simulink model "MLIinverter"  (R2019a)
settings: Solver=VariableStepAuto  StartTime=0.0  StopTime=10.0  RelTol=1e-3
libraries: powerlib x47, powerlib_meascontrol x15
settings Model: Creator=Administrator  LastModifiedBy=Administrator

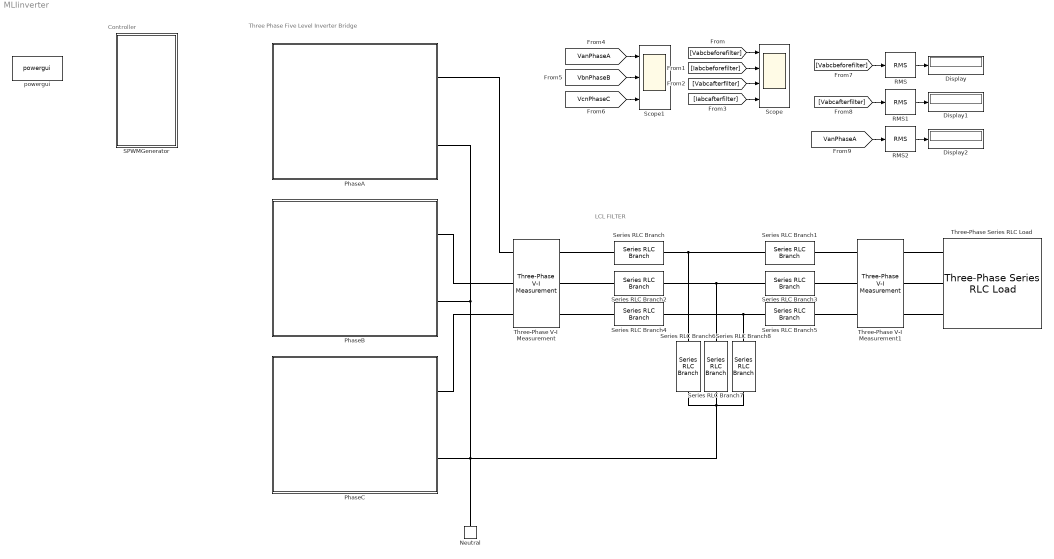
== system MLIinverter ==
  note: LCL FILTER
  note: Controller
  note: Three Phase Five Level Inverter Bridge
  Display : Display
  Display1 : Display
  Display2 : Display
  Neutral : powerlib/Elements/Neutral  LConnTagsString=a  NodeNumber=10
      settings: SourceProductName=Simscape Electrical  SourceProductBaseCode=PS
  PhaseA : Subsystem
  PhaseB : Subsystem
  PhaseC : Subsystem
  RMS : powerlib_meascontrol/Measurements/RMS  TrueRMS=on  Freq=50  RMSInit=0  Ts=0
      settings: SourceProductName=Simscape Electrical
  RMS1 : powerlib_meascontrol/Measurements/RMS  TrueRMS=on  Freq=50  RMSInit=0  Ts=0
      settings: SourceProductName=Simscape Electrical
  RMS2 : powerlib_meascontrol/Measurements/RMS  TrueRMS=on  Freq=50  RMSInit=0  Ts=0
      settings: SourceProductName=Simscape Electrical
  SPWMGenerator : Subsystem
  Scope : Scope  NumInputPorts=4
  Scope1 : Scope  NumInputPorts=3
  Series RLC Branch : powerlib/Elements/Series RLC Branch  LConnTagsString=__new0  RConnTagsString=__new0  BranchType=L  Resistance=1  Inductance=260e-3  SetiL0=off  InitialCurrent=0  Capacitance=1e-6  Setx0=off  InitialVoltage=0  Measurements=None
      settings: SourceProductName=Simscape Electrical
  Series RLC Branch1 : powerlib/Elements/Series RLC Branch  LConnTagsString=__new0  RConnTagsString=__new0  BranchType=L  Resistance=1  Inductance=14e-3  SetiL0=off  InitialCurrent=0  Capacitance=1e-6  Setx0=off  InitialVoltage=0  Measurements=None
      settings: SourceProductName=Simscape Electrical
  Series RLC Branch2 : powerlib/Elements/Series RLC Branch  LConnTagsString=__new0  RConnTagsString=__new0  BranchType=L  Resistance=1  Inductance=260e-3  SetiL0=off  InitialCurrent=0  Capacitance=1e-6  Setx0=off  InitialVoltage=0  Measurements=None
      settings: SourceProductName=Simscape Electrical
  Series RLC Branch3 : powerlib/Elements/Series RLC Branch  LConnTagsString=__new0  RConnTagsString=__new0  BranchType=L  Resistance=1  Inductance=14e-3  SetiL0=off  InitialCurrent=0  Capacitance=1e-6  Setx0=off  InitialVoltage=0  Measurements=None
      settings: SourceProductName=Simscape Electrical
  Series RLC Branch4 : powerlib/Elements/Series RLC Branch  LConnTagsString=__new0  RConnTagsString=__new0  BranchType=L  Resistance=1  Inductance=260e-3  SetiL0=off  InitialCurrent=0  Capacitance=1e-6  Setx0=off  InitialVoltage=0  Measurements=None
      settings: SourceProductName=Simscape Electrical
  Series RLC Branch5 : powerlib/Elements/Series RLC Branch  LConnTagsString=__new0  RConnTagsString=__new0  BranchType=L  Resistance=1  Inductance=14e-3  SetiL0=off  InitialCurrent=0  Capacitance=1e-6  Setx0=off  InitialVoltage=0  Measurements=None
      settings: SourceProductName=Simscape Electrical
  Series RLC Branch6 : powerlib/Elements/Series RLC Branch  LConnTagsString=__new0  RConnTagsString=__new0  BranchType=C  Resistance=1  Inductance=1e-3  SetiL0=off  InitialCurrent=0  Capacitance=18e-6  Setx0=off  InitialVoltage=0  Measurements=None
      settings: SourceProductName=Simscape Electrical
  Series RLC Branch7 : powerlib/Elements/Series RLC Branch  LConnTagsString=__new0  RConnTagsString=__new0  BranchType=C  Resistance=1  Inductance=1e-3  SetiL0=off  InitialCurrent=0  Capacitance=18e-6  Setx0=off  InitialVoltage=0  Measurements=None
      settings: SourceProductName=Simscape Electrical
  Series RLC Branch8 : powerlib/Elements/Series RLC Branch  LConnTagsString=__new0  RConnTagsString=__new0  BranchType=C  Resistance=1  Inductance=1e-3  SetiL0=off  InitialCurrent=0  Capacitance=18e-6  Setx0=off  InitialVoltage=0  Measurements=None
      settings: SourceProductName=Simscape Electrical
  Three-Phase Series RLC Load : powerlib/Elements/Three-Phase Series RLC Load  LConnTagsString=A|B|C  Configuration=Y (grounded)  NominalVoltage=400  Vabc=[1e3 1e3 1e3]  Vabcp=[1e3 1e3 1e3]  NominalFrequency=50  UnbalancedPower=off  ActivePower=1e3  InductivePower=0  CapacitivePower=0  Pabc=[10e3 9e3 11e3]  QLabc=[100 90 110]  QCabc=[100 90 110]  Pabcp=[10e3 9e3 11e3]  QLabcp=[100 90 110]  QCabcp=[100 90 110]  Measurements=None  LoadType=constant PQ
      settings: SourceProductName=Simscape Electrical
  Three-Phase V-I Measurement : powerlib/Measurements/Three-Phase V-I Measurement  VoltageMeasurement=phase-to-phase  SetLabelV=on  LabelV=Vabcbeforefilter  Vpu=off  VpuLL=off  CurrentMeasurement=yes  SetLabelI=on  LabelI=Iabcbeforefilter  Ipu=off  Pbase=100e6  Vbase=500e3  OutputType=Complex  PhasorSimulation=off  PSBequivalent=0
      settings: SourceProductName=Simscape Electrical
  Three-Phase V-I Measurement1 : powerlib/Measurements/Three-Phase V-I Measurement  VoltageMeasurement=phase-to-phase  SetLabelV=on  LabelV=Vabcafterfilter  Vpu=off  VpuLL=off  CurrentMeasurement=yes  SetLabelI=on  LabelI=Iabcafterfilter  Ipu=off  Pbase=100e6  Vbase=500e3  OutputType=Complex  PhasorSimulation=off  PSBequivalent=0
      settings: SourceProductName=Simscape Electrical
  powergui : powerlib/powergui  Priority=1  SimulationMode=Discrete  SampleTime=6e-6  frequency=60  Iterations=50  frequencyindice=0  Pbase=100e6  ErrMax=1e-4  UnitsV=kV  UnitsW=MW  buscounter=0  FunctionMessages=off  echomessages=off  EnableUseOfTLC=off  CurrentSourceSwitches=off  DisableSnubberDevices=off  DisableRonSwitches=off  DisableVfSwitches=off  DisplayEquations=off  AutomaticDiscreteSolvers=off  SolverType=Tustin/Backward Euler (TBE)  Interpol=off  ExternalGateDelay=off  methode=off  Ts=100  x0status=blocks  SPID=on  SwTol=0  HookPort=off  NonlinearTolerance=0  nMaxIteration=15  ContinueOnMaxIteration=off  RestoreLinks=warning  ResistiveCurrentMeasurement=off  Frange=[0:2:500]  Ylog=off  Xlog=on  ShowGrid=off  save=off  variable=ZData  structure=0  ZoomFFT=off  StartTime=0.0  cycles=1  DisplayStyle=1  fundamental=60  FreqAxis=off  MaxFrequency=1000  frequencyindicesteady=1  RmsSteady=1  display=off
      settings: SourceProductName=Simscape Electrical
  wires:
  [Vabcbeforefilter] -> Scope/1
  [Iabcbeforefilter] -> Scope/2
  [Iabcafterfilter] -> Scope/4
  [Vabcafterfilter] -> Scope/3
  [VanPhaseA] -> Scope1/1
  [VbnPhaseB] -> Scope1/2
  [VcnPhaseC] -> Scope1/3
  RMS/1 -> Display/1
  RMS1/1 -> Display1/1
  RMS2/1 -> Display2/1
  [Vabcbeforefilter] -> RMS/1
  [Vabcafterfilter] -> RMS1/1
  [VanPhaseA] -> RMS2/1
  connections:
  PhaseA/RConn1 -- Three-Phase V-I Measurement/LConn1
  PhaseB/RConn1 -- Three-Phase V-I Measurement/LConn2
  PhaseC/RConn1 -- Three-Phase V-I Measurement/LConn3
  Series RLC Branch/LConn1 -- Three-Phase V-I Measurement/RConn1
  Three-Phase V-I Measurement/RConn3 -- Series RLC Branch4/LConn1
  Three-Phase V-I Measurement1/RConn1 -- Three-Phase Series RLC Load/LConn1
  Three-Phase V-I Measurement1/RConn2 -- Three-Phase Series RLC Load/LConn2
  Three-Phase V-I Measurement1/RConn3 -- Three-Phase Series RLC Load/LConn3
  Three-Phase V-I Measurement/RConn2 -- Series RLC Branch2/LConn1
  Series RLC Branch2/RConn1 -- Series RLC Branch7/LConn1 -- Series RLC Branch3/LConn1
  Series RLC Branch1/LConn1 -- Series RLC Branch6/LConn1 -- Series RLC Branch/RConn1
  Series RLC Branch4/RConn1 -- Series RLC Branch5/LConn1 -- Series RLC Branch8/LConn1
  Series RLC Branch3/RConn1 -- Three-Phase V-I Measurement1/LConn2
  Series RLC Branch1/RConn1 -- Three-Phase V-I Measurement1/LConn1
  Three-Phase V-I Measurement1/LConn3 -- Series RLC Branch5/RConn1
  PhaseA/RConn2 -- PhaseB/RConn2 -- Series RLC Branch8/RConn1 -- Series RLC Branch7/RConn1 -- Series RLC Branch6/RConn1 -- Neutral/LConn1 -- PhaseC/RConn2

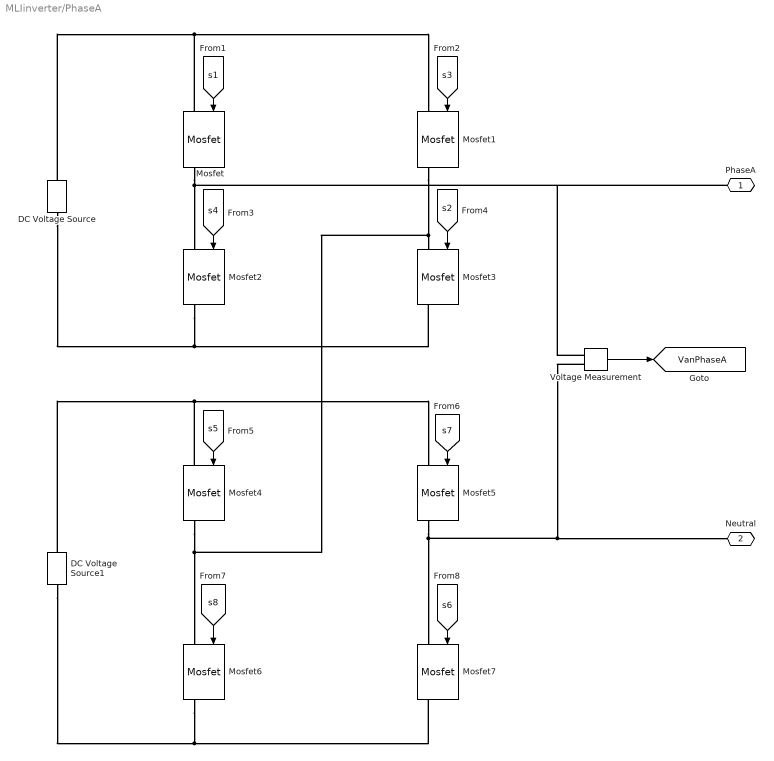
== system MLIinverter/PhaseA ==
  DC Voltage Source : powerlib/Electrical Sources/DC Voltage Source  Amplitude=160  Measurements=None
      settings: SourceProductName=Simscape Electrical
  DC Voltage Source1 : powerlib/Electrical Sources/DC Voltage Source  Amplitude=160  Measurements=None
      settings: SourceProductName=Simscape Electrical
  Mosfet{,1..7} (8 alike) : powerlib/Power Electronics/Mosfet  Ron=0.1  Lon=0  Rd=0.01  Vfd=0  IC=0  Rs=1e5  Cs=inf  Measurements=on
      settings: SourceProductName=Simscape Electrical
  Voltage Measurement : powerlib/Measurements/Voltage Measurement  PhasorSimulation=off  OutputType=Complex  PSBequivalent=0
      settings: SourceProductName=Simscape Electrical
  PhaseA : PMIOPort  Side=Right
  Neutral : PMIOPort  Port=2  Side=Right
  tag scope: VanPhaseA=global
  wires:
  [s2] -> Mosfet3/1
  Voltage Measurement/1 -> [VanPhaseA]
  [s4] -> Mosfet2/1
  [s6] -> Mosfet7/1
  [s7] -> Mosfet5/1
  [s8] -> Mosfet6/1
  [s1] -> Mosfet/1
  [s3] -> Mosfet1/1
  [s5] -> Mosfet4/1
  connections:
  Mosfet/RConn1 -- PhaseA/RConn1 -- Voltage Measurement/LConn1 -- Mosfet2/LConn1
  Mosfet6/RConn1 -- DC Voltage Source1/LConn1 -- Mosfet7/RConn1
  Mosfet2/RConn1 -- DC Voltage Source/LConn1 -- Mosfet3/RConn1
  Mosfet4/LConn1 -- DC Voltage Source1/RConn1 -- Mosfet5/LConn1
  Voltage Measurement/LConn2 -- Mosfet7/LConn1 -- Mosfet5/RConn1 -- Neutral/RConn1
  Mosfet/LConn1 -- DC Voltage Source/RConn1 -- Mosfet1/LConn1
  Mosfet1/RConn1 -- Mosfet6/LConn1 -- Mosfet4/RConn1 -- Mosfet3/LConn1

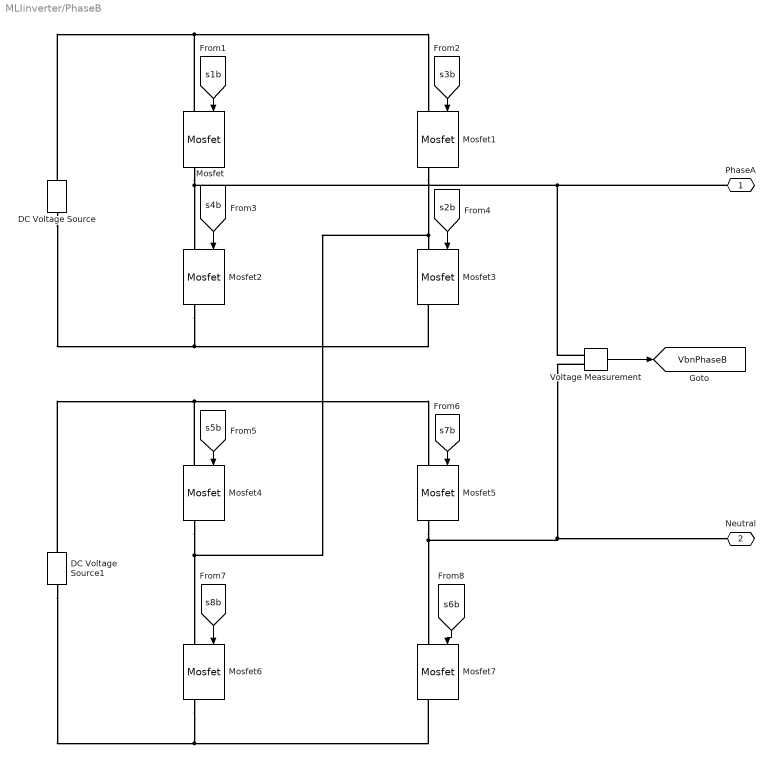
== system MLIinverter/PhaseB ==
  DC Voltage Source : powerlib/Electrical Sources/DC Voltage Source  Amplitude=160  Measurements=None
      settings: SourceProductName=Simscape Electrical
  DC Voltage Source1 : powerlib/Electrical Sources/DC Voltage Source  Amplitude=160  Measurements=None
      settings: SourceProductName=Simscape Electrical
  Mosfet{,1..7} (8 alike) : powerlib/Power Electronics/Mosfet  Ron=0.1  Lon=0  Rd=0.01  Vfd=0  IC=0  Rs=1e5  Cs=inf  Measurements=on
      settings: SourceProductName=Simscape Electrical
  Voltage Measurement : powerlib/Measurements/Voltage Measurement  PhasorSimulation=off  OutputType=Complex  PSBequivalent=0
      settings: SourceProductName=Simscape Electrical
  PhaseA : PMIOPort  Side=Right
  Neutral : PMIOPort  Port=2  Side=Right
  tag scope: VbnPhaseB=global
  wires:
  [s5b] -> Mosfet4/1
  [s3b] -> Mosfet1/1
  [s1b] -> Mosfet/1
  [s8b] -> Mosfet6/1
  [s7b] -> Mosfet5/1
  [s6b] -> Mosfet7/1
  [s4b] -> Mosfet2/1
  Voltage Measurement/1 -> [VbnPhaseB]
  [s2b] -> Mosfet3/1
  connections:
  DC Voltage Source/RConn1 -- Mosfet/LConn1 -- Mosfet1/LConn1
  Voltage Measurement/LConn2 -- Mosfet7/LConn1 -- Mosfet5/RConn1 -- Neutral/RConn1
  DC Voltage Source1/RConn1 -- Mosfet4/LConn1 -- Mosfet5/LConn1
  Mosfet1/RConn1 -- Mosfet6/LConn1 -- Mosfet4/RConn1 -- Mosfet3/LConn1
  DC Voltage Source/LConn1 -- Mosfet2/RConn1 -- Mosfet3/RConn1
  DC Voltage Source1/LConn1 -- Mosfet7/RConn1 -- Mosfet6/RConn1
  PhaseA/RConn1 -- Mosfet2/LConn1 -- Mosfet/RConn1 -- Voltage Measurement/LConn1

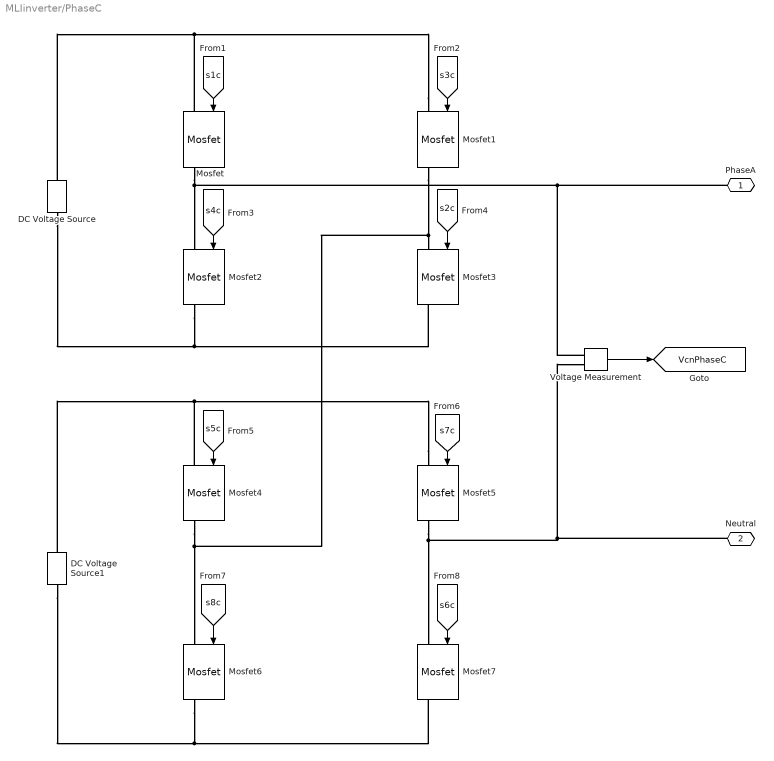
== system MLIinverter/PhaseC ==
  DC Voltage Source : powerlib/Electrical Sources/DC Voltage Source  Amplitude=160  Measurements=None
      settings: SourceProductName=Simscape Electrical
  DC Voltage Source1 : powerlib/Electrical Sources/DC Voltage Source  Amplitude=160  Measurements=None
      settings: SourceProductName=Simscape Electrical
  Mosfet{,1..7} (8 alike) : powerlib/Power Electronics/Mosfet  Ron=0.1  Lon=0  Rd=0.01  Vfd=0  IC=0  Rs=1e5  Cs=inf  Measurements=on
      settings: SourceProductName=Simscape Electrical
  Voltage Measurement : powerlib/Measurements/Voltage Measurement  PhasorSimulation=off  OutputType=Complex  PSBequivalent=0
      settings: SourceProductName=Simscape Electrical
  PhaseA : PMIOPort  Side=Right
  Neutral : PMIOPort  Port=2  Side=Right
  tag scope: VcnPhaseC=global
  wires:
  [s2c] -> Mosfet3/1
  Voltage Measurement/1 -> [VcnPhaseC]
  [s4c] -> Mosfet2/1
  [s6c] -> Mosfet7/1
  [s7c] -> Mosfet5/1
  [s8c] -> Mosfet6/1
  [s1c] -> Mosfet/1
  [s3c] -> Mosfet1/1
  [s5c] -> Mosfet4/1
  connections:
  Voltage Measurement/LConn1 -- Mosfet/RConn1 -- Mosfet2/LConn1 -- PhaseA/RConn1
  Mosfet6/RConn1 -- Mosfet7/RConn1 -- DC Voltage Source1/LConn1
  Mosfet3/RConn1 -- Mosfet2/RConn1 -- DC Voltage Source/LConn1
  Mosfet5/LConn1 -- Mosfet4/LConn1 -- DC Voltage Source1/RConn1
  Neutral/RConn1 -- Mosfet7/LConn1 -- Mosfet5/RConn1 -- Voltage Measurement/LConn2
  Mosfet1/LConn1 -- Mosfet/LConn1 -- DC Voltage Source/RConn1
  Mosfet1/RConn1 -- Mosfet6/LConn1 -- Mosfet4/RConn1 -- Mosfet3/LConn1

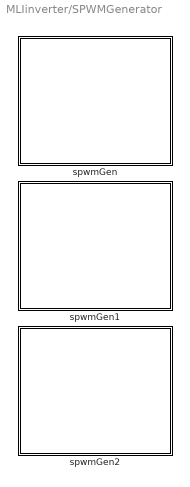
== system MLIinverter/SPWMGenerator ==
  spwmGen : Subsystem
  spwmGen1 : Subsystem
  spwmGen2 : Subsystem

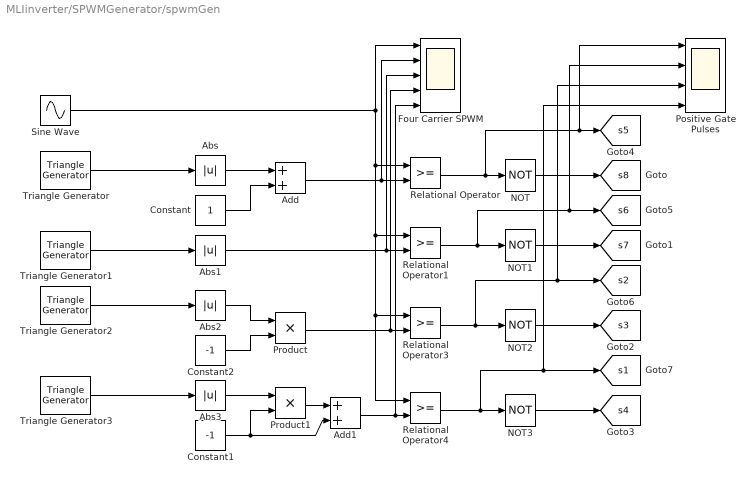
== system MLIinverter/SPWMGenerator/spwmGen ==
  Abs{,1..3} (4 alike) : Abs
  Add : Sum
  Add1 : Sum
  Constant : Constant
  Constant1 : Constant  Value=-1
  Constant2 : Constant  Value=-1
  Four Carrier SPWM : Scope  NumInputPorts=5
  NOT{,1..3} (4 alike) : Logic  Operator=NOT  IconShape=distinctive  AllPortsSameDT=off  OutDataTypeStr=boolean
  Positive Gate Pulses : Scope  NumInputPorts=4
  Product : Product
  Product1 : Product
  Relational Operator{,1,3..4} (4 alike) : RelationalOperator  OutDataTypeStr=boolean  RndMeth=Simplest
  Sine Wave : Sin  Amplitude=2  Frequency=2*pi*50  SampleTime=0
  Triangle Generator : powerlib_meascontrol/Pulse & Signal Generators/Triangle Generator  Freq=10e3  Phase=90  Ts=0
      settings: SourceProductName=Simscape Electrical
  Triangle Generator1 : powerlib_meascontrol/Pulse & Signal Generators/Triangle Generator  Freq=10e3  Phase=90  Ts=0
      settings: SourceProductName=Simscape Electrical
  Triangle Generator2 : powerlib_meascontrol/Pulse & Signal Generators/Triangle Generator  Freq=10e3  Phase=0  Ts=0
      settings: SourceProductName=Simscape Electrical
  Triangle Generator3 : powerlib_meascontrol/Pulse & Signal Generators/Triangle Generator  Freq=10e3  Phase=0  Ts=0
      settings: SourceProductName=Simscape Electrical
  tag scope: s1=global, s2=global, s3=global, s4=global, s5=global, s6=global, s7=global, s8=global
  wires:
  Product1/1 -> Add1/1
  Add1/1 -> Four Carrier SPWM/5, Relational Operator4/2
  NOT3/1 -> [s4]
  Sine Wave/1 -> Four Carrier SPWM/1, Relational Operator/1, Relational Operator4/1, Relational Operator3/1, Relational Operator1/1
  Triangle Generator/1 -> Abs/1
  Constant1/1 -> Add1/2, Product1/2
  Relational Operator/1 -> Positive Gate Pulses/1, [s5], NOT/1
  Add/1 -> Relational Operator/2, Four Carrier SPWM/2
  NOT/1 -> [s8]
  Abs3/1 -> Product1/1
  Abs/1 -> Add/1
  NOT1/1 -> [s7]
  Relational Operator3/1 -> Positive Gate Pulses/3, [s2], NOT2/1
  Abs1/1 -> Relational Operator1/2, Four Carrier SPWM/3
  NOT2/1 -> [s3]
  Product/1 -> Relational Operator3/2, Four Carrier SPWM/4
  Relational Operator1/1 -> Positive Gate Pulses/2, [s6], NOT1/1
  Relational Operator4/1 -> Positive Gate Pulses/4, [s1], NOT3/1
  Triangle Generator3/1 -> Abs3/1
  Triangle Generator1/1 -> Abs1/1
  Constant/1 -> Add/2
  Triangle Generator2/1 -> Abs2/1
  Abs2/1 -> Product/1
  Constant2/1 -> Product/2

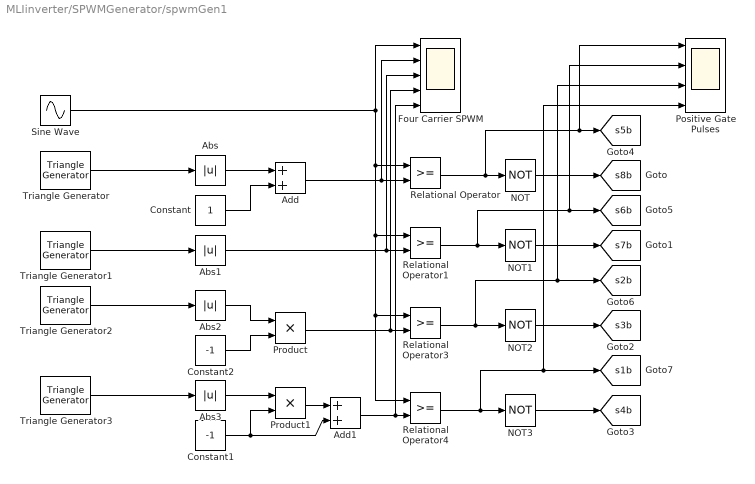
== system MLIinverter/SPWMGenerator/spwmGen1 ==
  Abs{,1..3} (4 alike) : Abs
  Add : Sum
  Add1 : Sum
  Constant : Constant
  Constant1 : Constant  Value=-1
  Constant2 : Constant  Value=-1
  Four Carrier SPWM : Scope  NumInputPorts=5
  NOT{,1..3} (4 alike) : Logic  Operator=NOT  IconShape=distinctive  AllPortsSameDT=off  OutDataTypeStr=boolean
  Positive Gate Pulses : Scope  NumInputPorts=4
  Product : Product
  Product1 : Product
  Relational Operator{,1,3..4} (4 alike) : RelationalOperator  OutDataTypeStr=boolean  RndMeth=Simplest
  Sine Wave : Sin  Amplitude=2  Frequency=2*pi*50  Phase=2*pi/3  SampleTime=0
  Triangle Generator : powerlib_meascontrol/Pulse & Signal Generators/Triangle Generator  Freq=10e3  Phase=90  Ts=0
      settings: SourceProductName=Simscape Electrical
  Triangle Generator1 : powerlib_meascontrol/Pulse & Signal Generators/Triangle Generator  Freq=10e3  Phase=90  Ts=0
      settings: SourceProductName=Simscape Electrical
  Triangle Generator2 : powerlib_meascontrol/Pulse & Signal Generators/Triangle Generator  Freq=10e3  Phase=0  Ts=0
      settings: SourceProductName=Simscape Electrical
  Triangle Generator3 : powerlib_meascontrol/Pulse & Signal Generators/Triangle Generator  Freq=10e3  Phase=0  Ts=0
      settings: SourceProductName=Simscape Electrical
  tag scope: s1b=global, s2b=global, s3b=global, s4b=global, s5b=global, s6b=global, s7b=global, s8b=global
  wires:
  Constant2/1 -> Product/2
  Abs2/1 -> Product/1
  Triangle Generator2/1 -> Abs2/1
  Constant/1 -> Add/2
  Triangle Generator1/1 -> Abs1/1
  Triangle Generator3/1 -> Abs3/1
  Relational Operator4/1 -> NOT3/1, [s1b], Positive Gate Pulses/4
  Relational Operator1/1 -> NOT1/1, [s6b], Positive Gate Pulses/2
  Product/1 -> Four Carrier SPWM/4, Relational Operator3/2
  NOT2/1 -> [s3b]
  Abs1/1 -> Four Carrier SPWM/3, Relational Operator1/2
  Relational Operator3/1 -> NOT2/1, [s2b], Positive Gate Pulses/3
  NOT1/1 -> [s7b]
  Abs/1 -> Add/1
  Abs3/1 -> Product1/1
  NOT/1 -> [s8b]
  Add/1 -> Four Carrier SPWM/2, Relational Operator/2
  Relational Operator/1 -> NOT/1, [s5b], Positive Gate Pulses/1
  Constant1/1 -> Product1/2, Add1/2
  Triangle Generator/1 -> Abs/1
  Sine Wave/1 -> Relational Operator1/1, Relational Operator3/1, Relational Operator4/1, Relational Operator/1, Four Carrier SPWM/1
  NOT3/1 -> [s4b]
  Add1/1 -> Relational Operator4/2, Four Carrier SPWM/5
  Product1/1 -> Add1/1

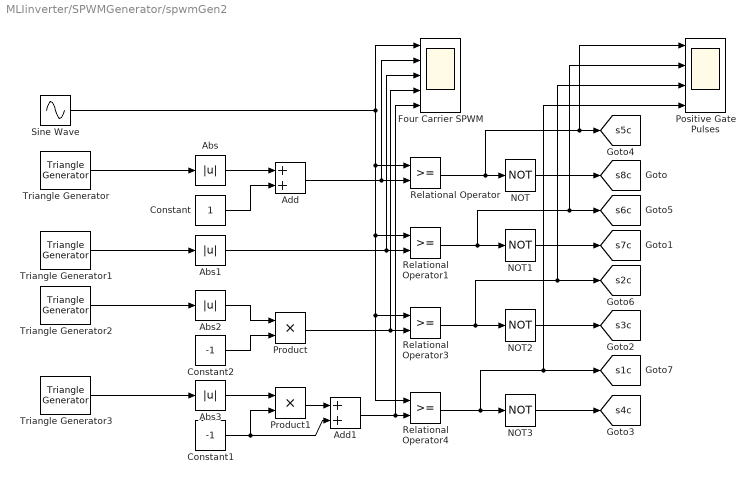
== system MLIinverter/SPWMGenerator/spwmGen2 ==
  Abs{,1..3} (4 alike) : Abs
  Add : Sum
  Add1 : Sum
  Constant : Constant
  Constant1 : Constant  Value=-1
  Constant2 : Constant  Value=-1
  Four Carrier SPWM : Scope  NumInputPorts=5
  NOT{,1..3} (4 alike) : Logic  Operator=NOT  IconShape=distinctive  AllPortsSameDT=off  OutDataTypeStr=boolean
  Positive Gate Pulses : Scope  NumInputPorts=4
  Product : Product
  Product1 : Product
  Relational Operator{,1,3..4} (4 alike) : RelationalOperator  OutDataTypeStr=boolean  RndMeth=Simplest
  Sine Wave : Sin  Amplitude=2  Frequency=2*pi*50  Phase=4*pi/3  SampleTime=0
  Triangle Generator : powerlib_meascontrol/Pulse & Signal Generators/Triangle Generator  Freq=10e3  Phase=90  Ts=0
      settings: SourceProductName=Simscape Electrical
  Triangle Generator1 : powerlib_meascontrol/Pulse & Signal Generators/Triangle Generator  Freq=10e3  Phase=90  Ts=0
      settings: SourceProductName=Simscape Electrical
  Triangle Generator2 : powerlib_meascontrol/Pulse & Signal Generators/Triangle Generator  Freq=10e3  Phase=0  Ts=0
      settings: SourceProductName=Simscape Electrical
  Triangle Generator3 : powerlib_meascontrol/Pulse & Signal Generators/Triangle Generator  Freq=10e3  Phase=0  Ts=0
      settings: SourceProductName=Simscape Electrical
  tag scope: s1c=global, s2c=global, s3c=global, s4c=global, s5c=global, s6c=global, s7c=global, s8c=global
  wires:
  Product1/1 -> Add1/1
  Add1/1 -> Four Carrier SPWM/5, Relational Operator4/2
  NOT3/1 -> [s4c]
  Sine Wave/1 -> Four Carrier SPWM/1, Relational Operator/1, Relational Operator4/1, Relational Operator3/1, Relational Operator1/1
  Triangle Generator/1 -> Abs/1
  Constant1/1 -> Add1/2, Product1/2
  Relational Operator/1 -> Positive Gate Pulses/1, [s5c], NOT/1
  Add/1 -> Relational Operator/2, Four Carrier SPWM/2
  NOT/1 -> [s8c]
  Abs3/1 -> Product1/1
  Abs/1 -> Add/1
  NOT1/1 -> [s7c]
  Relational Operator3/1 -> Positive Gate Pulses/3, [s2c], NOT2/1
  Abs1/1 -> Relational Operator1/2, Four Carrier SPWM/3
  NOT2/1 -> [s3c]
  Product/1 -> Relational Operator3/2, Four Carrier SPWM/4
  Relational Operator1/1 -> Positive Gate Pulses/2, [s6c], NOT1/1
  Relational Operator4/1 -> Positive Gate Pulses/4, [s1c], NOT3/1
  Triangle Generator3/1 -> Abs3/1
  Triangle Generator1/1 -> Abs1/1
  Constant/1 -> Add/2
  Triangle Generator2/1 -> Abs2/1
  Abs2/1 -> Product/1
  Constant2/1 -> Product/2
